simulink model "testRPiSerialFrameRx"  (R2016a)
settings: Solver=FixedStepAuto  StartTime=0.0  StopTime=inf  FixedStep=0.7  RelTol=1e-3
libraries: RPi x1
settings Model: SimulationMode=external  Creator=user  LastModifiedBy=user
settings SolverCC: PositivePriorityOrder=on
settings OptimizationCC: OptimizeModelRefInitCode=on  LifeSpan=1  MaxStackSize=64
settings HardwareCC: ProdBitPerPointer=32  ProdLargestAtomicInteger=Long  ProdLargestAtomicFloat=Double  ProdWordSize=32  ProdHWDeviceType=ARM Compatible->ARM Cortex
settings RTWCC: SystemTargetFile=ert.tlc  HardwareBoard=Raspberry Pi  TemplateMakefile=ert_default_tmf  GenerateReport=on  Toolchain=GNU GCC Raspberry Pi  IncludeHyperlinkInReport=on  LaunchReport=on  GenerateTraceInfo=on  GenerateTraceReport=on  GenerateTraceReportSl=on  GenerateTraceReportSf=on  GenerateTraceReportEml=on
settings CodeAppCC: ForceParamTrailComments=on  IgnoreCustomStorageClasses=off  OperatorAnnotations=on  SimulinkDataObjDesc=on  SFDataObjDesc=on  MATLABFcnDesc=on  InsertBlockDesc=on  MATLABSourceComments=on
settings ERTTargetCC: SupportVariableSizeSignals=on

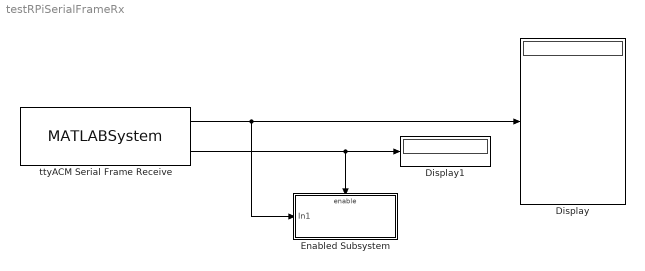
== system testRPiSerialFrameRx ==
  Display : Display
  Display1 : Display
  Enabled Subsystem : Subsystem  TreatAsAtomicUnit=on
  ttyACM Serial Frame Receive : MATLABSystem  System=rpiACMserialFrameRxClass  portID=0  SOFbyte=254  EOFbyte=255  msgLen=4  SimulateUsing=Code generation
      mask Type: rpiACMserialFrameRxClass
      mask Display:
      | disp('rpiACMserialFrameRxClass');
      | port_label('output',1,'buffer');
      | port_label('output',2,'status');
  wires:
  ttyACM Serial Frame Receive/2 -> Enabled Subsystem/Enable, Display1/1
  ttyACM Serial Frame Receive/1 -> Enabled Subsystem/1(In1), Display/1

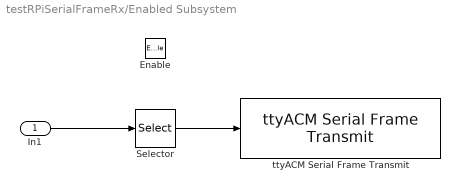
== system testRPiSerialFrameRx/Enabled Subsystem ==
  In1 : Inport
  Enable : EnablePort
  Selector : Selector  InputPortWidth=4  IndexOptions=Index vector (dialog)  Indices=[1]  OutputSizes=1
  ttyACM Serial Frame Transmit : RPi/ttyACM Serial Frame Transmit  portID=0  SOFbyte=254  EOFbyte=255  SimulateUsing=Code generation
  wires:
  In1/1 -> Selector/1
  Selector/1 -> ttyACM Serial Frame Transmit/1
